simulink model "Final_Design"  (R2017b)
settings: Solver=VariableStepAuto  StartTime=0.0  StopTime=150  RelTol=1e-3
libraries: xbsIndex_r4 x23
settings Model: Creator=the20  LastModifiedBy=the20

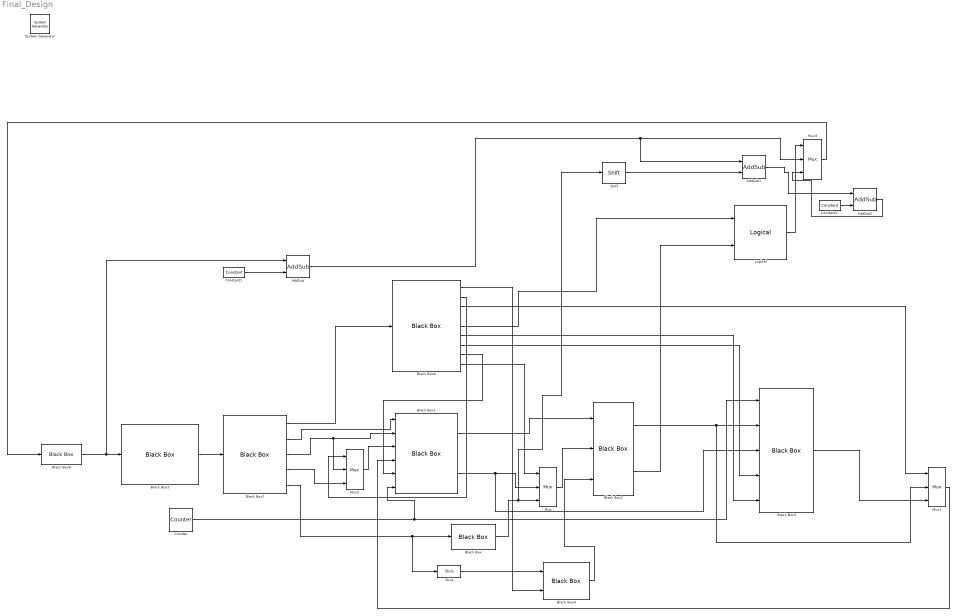
== system Final_Design ==
  " System Generator" : xbsIndex_r4/ System Generator  Tag=genX  xilinxfamily=kintex7  part=xc7k325t  speed=-3  package=fbg676  synthesis_tool=Vivado  clock_wrapper=Clock Enables  directory=./netlist  proj_type=Vivado  Synth_file=Vivado Synthesis Defaults  Impl_file=Vivado Implementation Defaults  testbench=off  simulink_period=1  sysclk_period=10  dcm_input_clock_period=10  incr_netlist=off  trim_vbits=Everywhere in SubSystem  dbl_ovrd=According to Block Masks  core_generation=According to Block Masks  run_coregen=off  deprecated_control=off  eval_field=0  block_type=sysgen
  AddSub : xbsIndex_r4/AddSub  mode=Addition  use_carryin=off  use_carryout=off  en=off  latency=0  precision=User Defined  arith_type=Unsigned  n_bits=32  bin_pt=0  quantization=Truncate  overflow=Wrap  use_behavioral_HDL=off  hw_selection=Fabric  pipelined=off  dbl_ovrd=off  block_type=addsub
  AddSub1 : xbsIndex_r4/AddSub  mode=Addition  use_carryin=off  use_carryout=off  en=off  latency=0  precision=User Defined  arith_type="Signed  (2's comp)"  n_bits=32  bin_pt=0  quantization=Truncate  overflow=Wrap  use_behavioral_HDL=off  hw_selection=Fabric  pipelined=off  dbl_ovrd=off  block_type=addsub
  AddSub2 : xbsIndex_r4/AddSub  mode=Subtraction  use_carryin=off  use_carryout=off  en=off  latency=0  precision=User Defined  arith_type="Signed  (2's comp)"  n_bits=32  bin_pt=0  quantization=Truncate  overflow=Wrap  use_behavioral_HDL=off  hw_selection=Fabric  pipelined=off  dbl_ovrd=off  block_type=addsub
  Black Box : xbsIndex_r4/Black Box  init_code=Sign_Extender_config  sim_method=ISE Simulator  verbose=off  block_type=blackbox2
  Black Box1 : xbsIndex_r4/Black Box  init_code=regFile_config  sim_method=ISE Simulator  verbose=off  block_type=blackbox2
  Black Box2 : xbsIndex_r4/Black Box  init_code=mipsalu_config  sim_method=ISE Simulator  verbose=off  block_type=blackbox2
  Black Box3 : xbsIndex_r4/Black Box  init_code=Data_Memory_config  sim_method=ISE Simulator  verbose=off  block_type=blackbox2
  Black Box4 : xbsIndex_r4/Black Box  init_code=ALU_Control_config  sim_method=ISE Simulator  verbose=off  block_type=blackbox2
  Black Box5 : xbsIndex_r4/Black Box  init_code=InstructionMemory_config  sim_method=ISE Simulator  verbose=off  block_type=blackbox2
  Black Box6 : xbsIndex_r4/Black Box  init_code=Control_Unit_config  sim_method=ISE Simulator  verbose=off  block_type=blackbox2
  Black Box7 : xbsIndex_r4/Black Box  init_code=Bit_Slicer_config  sim_method=ISE Simulator  verbose=off  block_type=blackbox2
  Black Box8 : xbsIndex_r4/Black Box  init_code=PC_config  sim_method=ISE Simulator  verbose=off  block_type=blackbox2
  Constant1 : xbsIndex_r4/Constant  const=4  gui_display_data_type=Fixed-point  arith_type=Unsigned  n_bits=32  bin_pt=0  preci_type=Single  exp_width=8  frac_width=24  explicit_period=on  period=1  equ=P=C  opselect=C  inp2=PCIN>>17  opr=+  inp1=P  carry=CIN  dbl_ovrd=off  block_type=constant
  Constant2 : xbsIndex_r4/Constant  const=4  gui_display_data_type=Fixed-point  arith_type=Signed (2's comp)  n_bits=32  bin_pt=0  preci_type=Single  exp_width=8  frac_width=24  explicit_period=on  period=1  equ=P=C  opselect=C  inp2=PCIN>>17  opr=+  inp1=P  carry=CIN  dbl_ovrd=off  block_type=constant
  Counter : xbsIndex_r4/Counter  cnt_type=Free Running  cnt_to=Inf  operation=Up  start_count=0  cnt_by_val=1  arith_type=Unsigned  n_bits=1  bin_pt=0  load_pin=off  rst=off  en=off  explicit_period=on  period=1  use_behavioral_HDL=off  implementation=Fabric  dbl_ovrd=off  block_type=counter
  Logical : xbsIndex_r4/Logical  logical_function=AND  inputs=2  en=off  latency=0  precision=Full  arith_type=Unsigned  n_bits=16  bin_pt=0  align_bp=on  dbl_ovrd=off  block_type=logical
  Mux : xbsIndex_r4/Mux  inputs=2  en=off  latency=0  precision=Full  arith_type=Unsigned  n_bits=16  bin_pt=14  quantization=Truncate  overflow=Wrap  dbl_ovrd=off  block_type=mux
  Mux1 : xbsIndex_r4/Mux  inputs=2  en=off  latency=1  precision=Full  arith_type=Unsigned  n_bits=16  bin_pt=14  quantization=Truncate  overflow=Wrap  dbl_ovrd=off  block_type=mux
  Mux2 : xbsIndex_r4/Mux  inputs=2  en=off  latency=0  precision=Full  arith_type=Unsigned  n_bits=16  bin_pt=14  quantization=Truncate  overflow=Wrap  dbl_ovrd=off  block_type=mux
  Mux3 : xbsIndex_r4/Mux  inputs=2  en=off  latency=2  precision=User Defined  arith_type=Unsigned  n_bits=32  bin_pt=0  quantization=Truncate  overflow=Wrap  dbl_ovrd=off  block_type=mux
  Shift : xbsIndex_r4/Shift  shift_dir=Left  shift_bits=2  en=off  latency=0  precision=User Defined  arith_type=Unsigned  n_bits=32  bin_pt=0  quantization=Truncate  overflow=Wrap  dbl_ovrd=off  block_type=shift
  Slice : xbsIndex_r4/Slice  nbits=6  boolean_output=off  mode=Lower Bit Location + Width  bit1=0  base1=MSB of Input  bit0=0  base0=LSB of Input  dbl_ovrd=off  block_type=slice
  wires:
  Black Box7/5 -> Slice/1, Black Box/1
  Mux/1 -> Black Box2/2
  Black Box3/1 -> Mux1/3
  Black Box2/1 -> Black Box3/2, Mux1/2
  Mux1/1 -> Black Box1/4
  Black Box1/1 -> Black Box2/1
  Black Box4/1 -> Black Box2/3
  Slice/1 -> Black Box4/1
  Black Box5/1 -> Black Box7/1
  Black Box7/2 -> Black Box1/1
  Black Box7/3 -> Black Box1/2, Mux2/2
  Mux2/1 -> Black Box1/3
  Black Box7/4 -> Mux2/3
  Black Box7/1 -> Black Box6/1
  Black Box6/9 -> Mux/1
  Black Box6/8 -> Black Box1/5
  Black Box6/7 -> Black Box3/4
  Black Box6/6 -> Black Box3/5
  Black Box6/3 -> Mux1/1
  Black Box6/2 -> Mux2/1
  Black Box6/1 -> Black Box4/2
  Black Box1/2 -> Black Box3/3, Mux/2
  Counter/1 -> Black Box3/1, Black Box1/6
  AddSub/1 -> AddSub1/1, Mux3/2
  Constant1/1 -> AddSub/2
  Black Box/1 -> Mux/3, Shift/1
  AddSub1/1 -> AddSub2/1
  Black Box6/5 -> Logical/1
  Shift/1 -> AddSub1/2
  Logical/1 -> Mux3/1
  Black Box2/2 -> Logical/2
  Mux3/1 -> Black Box8/1
  Black Box8/1 -> AddSub/1, Black Box5/1
  AddSub2/1 -> Mux3/3
  Constant2/1 -> AddSub2/2
